simulink model "simulacion"  (R2015b)
settings: Solver=FixedStepAuto  StartTime=0.0  StopTime=10.0  FixedStep=1e-3  RelTol=1e-3
settings Model: Creator=Tomas  LastModifiedBy=Tomas

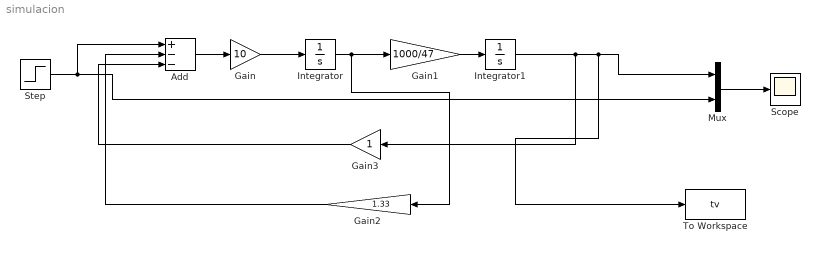
== system simulacion ==
  Add : Sum  Inputs=+--
  Gain : Gain  Gain=10
  Gain1 : Gain  Gain=1000/47
  Gain2 : Gain  Gain=1.33
  Gain3 : Gain
  Integrator : Integrator
  Integrator1 : Integrator
  Mux : Mux  Inputs=2
  Scope : Scope
  Step : Step  SampleTime=0
  To Workspace : ToWorkspace  VariableName=tv  SaveFormat=Structure With Time  SampleTime=-1
  wires:
  Mux/1 -> Scope/1
  Gain/1 -> Integrator/1
  Gain1/1 -> Integrator1/1
  Integrator/1 -> Gain2/1, Gain1/1
  Integrator1/1 -> Gain3/1, To Workspace/1, Mux/1
  Step/1 -> Add/1, Mux/2
  Add/1 -> Gain/1
  Gain3/1 -> Add/3
  Gain2/1 -> Add/2
